simulink model "ac3_example_MMCT"  (R2023a)
settings: Solver=FixedStepDiscrete  StartTime=0.0  StopTime=3  FixedStep=Ts  RelTol=1e-3  EnableMultiTasking=on
PreLoadFcn:
  | Ts = 2e-6;
undefined symbols (not defined in the file): DiscIntNeverNeededParam
libraries: simulink_extras x7, spsCurrentMeasurementLib x3, spsVoltageMeasurementLib x3, spsDrivesPrivateModels x2, spsStairGeneratorLib x2, spsThreePhaseSourceLib x1, spsDrivesDcBusModel x1, spsSpaceVectorModulatorLib x1, eeAdaptiveController x1, slctrlblks x1, simulink x1, slpidlib x1
(part 2 of 3)

== system ac3_example_MMCT/Field-Oriented Control Induction Motor Drive/F.O.C./Average/Teta Calculation ==
  note: wm= Rotor mechanical speed (rad/s)
  note: wr = Rotor frequency (rad/s) = Lm *Iq / ( Tr * Phir)
  note: Teta= Electrical angle= integ ( wr + wm)
  Iq : Inport
  Phir : Inport  Port=2
  wm : Inport  Port=3
  Discrete-Time Integrator : DiscreteIntegrator  IntegratorMethod=Integration: Trapezoidal  SampleTime=Tvect  ICPrevOutput=DiscIntNeverNeededParam  ICPrevScaledInput=DiscIntNeverNeededParam
  Fcn : Fcn  Expr=Lm*u[1]/(u[2]*(Lr/Rr))
  Gain2 : Gain  SaturateOnIntegerOverflow=on  OutDataTypeStr=Inherit: Same as input  ParamDataTypeStr=Inherit: Same as input
  Gain3 : Gain  Gain=p  SaturateOnIntegerOverflow=on  OutDataTypeStr=Inherit: Same as input  ParamDataTypeStr=Inherit: Same as input
  Mux : Mux  Inputs=2
  Saturation : Saturate  UpperLimit=inf  LowerLimit=1e-3
  Sum : Sum  InputSameDT=on  SaturateOnIntegerOverflow=on  OutDataTypeStr=Inherit: Same as first input
  Unit Delay5 : UnitDelay  SampleTime=Tvect  HasFrameUpgradeWarning=on
  Thetae : Outport  InitialOutput=0  VectorParamsAs1DForOutWhenUnconnected=off
  we : Outport  Port=2  InitialOutput=0  VectorParamsAs1DForOutWhenUnconnected=off
  wires:
  Fcn/1 -> Gain2/1
  wm/1 -> Gain3/1
  Gain2/1 -> Sum/1
  Gain3/1 -> Sum/2
  Sum/1 -> we/1, Discrete-Time Integrator/1
  Discrete-Time Integrator/1 -> Thetae/1
  Unit Delay5/1 -> Mux/1
  Saturation/1 -> Mux/2
  Mux/1 -> Fcn/1
  Iq/1 -> Unit Delay5/1
  Phir/1 -> Saturation/1

== system ac3_example_MMCT/Field-Oriented Control Induction Motor Drive/F.O.C./Average/id* Calculation ==
  note: Lm= 34.7 mH
  note: Id* = Phir*/ Lm
  Phir* : Inport
  KF : Gain  Gain=1/Lm  SaturateOnIntegerOverflow=on  OutDataTypeStr=Inherit: Same as input  ParamDataTypeStr=Inherit: Same as input
  Id* : Outport  VectorParamsAs1DForOutWhenUnconnected=off
  wires:
  Phir*/1 -> KF/1
  KF/1 -> Id*/1

== system ac3_example_MMCT/Field-Oriented Control Induction Motor Drive/F.O.C./Average/iqs* Calculation ==
  Te* : Inport
  Phir : Inport  Port=2
  Fcn : Fcn  Expr=(2/3)*(1/p)*(Lr/Lm)*u[1]/(u[2]+1e-3*0)
  Mux1 : Mux  Inputs=2
  Saturation : Saturate  UpperLimit=inf  LowerLimit=1e-3
  Iq* : Outport  InitialOutput=0  VectorParamsAs1DForOutWhenUnconnected=off
  wires:
  Saturation/1 -> Mux1/2
  Mux1/1 -> Fcn/1
  Te*/1 -> Mux1/1
  Fcn/1 -> Iq*/1
  Phir/1 -> Saturation/1

== system ac3_example_MMCT/Field-Oriented Control Induction Motor Drive/F.O.C./Detailed/ABC-DQ ==
  Teta : Inport
  Iabc : Inport  Port=2
  Fcn : Fcn  Expr=sin(u)
  Fcn1 : Fcn  Expr=cos(u)
  Gain : Gain  Gain=2/3  SaturateOnIntegerOverflow=on  OutDataTypeStr=Inherit: Same as input  ParamDataTypeStr=Inherit: Same as input
  Gain1 : Gain  Gain=2/3  SaturateOnIntegerOverflow=on  OutDataTypeStr=Inherit: Same as input  ParamDataTypeStr=Inherit: Same as input
  Mux : Mux  Inputs=[1 1 3]
  id : Fcn  Expr=u[1]*u[3]+(1.7320508*u[2]-u[1])*u[4]*0.5+(-u[1]-1.7320508*u[2])*u[5]*0.5
  iq : Fcn  Expr=-u[2]*u[3]+(u[2]+1.7320508*u[1])*u[4]*0.5+(u[2]-1.7320508*u[1])*u[5]*0.5
  Id : Outport  InitialOutput=0  VectorParamsAs1DForOutWhenUnconnected=off
  Iq : Outport  Port=2  InitialOutput=0  VectorParamsAs1DForOutWhenUnconnected=off
  wires:
  Gain1/1 -> Iq/1
  Gain/1 -> Id/1
  id/1 -> Gain/1
  iq/1 -> Gain1/1
  Iabc/1 -> Mux/3
  Mux/1 -> id/1, iq/1
  Teta/1 -> Fcn/1, Fcn1/1
  Fcn1/1 -> Mux/1
  Fcn/1 -> Mux/2

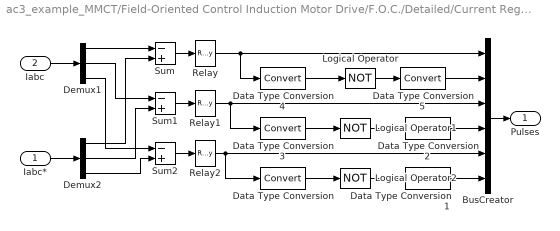
== system ac3_example_MMCT/Field-Oriented Control Induction Motor Drive/F.O.C./Detailed/Current Regulator ==
  Iabc* : Inport
  Iabc : Inport  Port=2
  BusCreator : BusCreator  Inputs=6
  Data Type Conversion{,1..5} (6 alike) : DataTypeConversion
  Demux1 : Demux  Outputs=3
      settings: DisplayOption=none
  Demux2 : Demux  Outputs=3
      settings: DisplayOption=none
  Logical Operator : Logic  Operator=NOT
  Logical Operator1 : Logic  Operator=NOT
  Logical Operator2 : Logic  Operator=NOT
  Relay : Relay  OnSwitchValue=h/2  OffSwitchValue=-h/2
  Relay1 : Relay  OnSwitchValue=h/2  OffSwitchValue=-h/2
  Relay2 : Relay  OnSwitchValue=h/2  OffSwitchValue=-h/2
  Sum : Sum  Inputs=-+  InputSameDT=on  SaturateOnIntegerOverflow=on  OutDataTypeStr=Inherit: Same as first input
  Sum1 : Sum  Inputs=-+  InputSameDT=on  SaturateOnIntegerOverflow=on  OutDataTypeStr=Inherit: Same as first input
  Sum2 : Sum  Inputs=-+  InputSameDT=on  SaturateOnIntegerOverflow=on  OutDataTypeStr=Inherit: Same as first input
  Pulses : Outport  InitialOutput=0  VectorParamsAs1DForOutWhenUnconnected=off
  wires:
  Logical Operator2/1 -> Data Type Conversion1/1
  Logical Operator1/1 -> Data Type Conversion2/1
  Logical Operator/1 -> Data Type Conversion5/1
  Relay2/1 -> BusCreator/5, Data Type Conversion/1
  Relay1/1 -> BusCreator/3, Data Type Conversion3/1
  Relay/1 -> BusCreator/1, Data Type Conversion4/1
  Iabc*/1 -> Demux2/1
  Demux2/1 -> Sum/2
  Demux2/2 -> Sum1/2
  Demux2/3 -> Sum2/2
  Demux1/3 -> Sum2/1
  Sum2/1 -> Relay2/1
  Iabc/1 -> Demux1/1
  BusCreator/1 -> Pulses/1
  Demux1/2 -> Sum1/1
  Demux1/1 -> Sum/1
  Sum1/1 -> Relay1/1
  Sum/1 -> Relay/1
  Data Type Conversion/1 -> Logical Operator2/1
  Data Type Conversion1/1 -> BusCreator/6
  Data Type Conversion2/1 -> BusCreator/4
  Data Type Conversion3/1 -> Logical Operator1/1
  Data Type Conversion4/1 -> Logical Operator/1
  Data Type Conversion5/1 -> BusCreator/2

== system ac3_example_MMCT/Field-Oriented Control Induction Motor Drive/F.O.C./Detailed/DQ-ABC ==
  Id* : Inport
  Iq* : Inport  Port=2
  Teta : Inport  Port=3
  Fcn : Fcn  Expr=sin(u)
  Fcn1 : Fcn  Expr=cos(u)
  Gain2 : Gain  SaturateOnIntegerOverflow=on  OutDataTypeStr=Inherit: Same as input  ParamDataTypeStr=Inherit: Same as input
  Gain3 : Gain  SaturateOnIntegerOverflow=on  OutDataTypeStr=Inherit: Same as input  ParamDataTypeStr=Inherit: Same as input
  Gain4 : Gain  SaturateOnIntegerOverflow=on  OutDataTypeStr=Inherit: Same as input  ParamDataTypeStr=Inherit: Same as input
  Mux : Mux
  Mux2 : Mux  Inputs=3
  ia : Fcn  Expr=-u[3]*u[2] + u[4]*u[1]
  ib : Fcn  Expr=(-u[1]+1.7320508*u[2])*u[4]*0.5+(u[2]+1.7320508*u[1])*u[3]*0.5
  ic : Sum  Inputs=--  InputSameDT=on  SaturateOnIntegerOverflow=on  OutDataTypeStr=Inherit: Same as first input
  Iabc* : Outport  InitialOutput=0  VectorParamsAs1DForOutWhenUnconnected=off
  wires:
  ib/1 -> ic/1, Gain3/1
  ia/1 -> ic/2, Gain2/1
  Gain2/1 -> Mux2/1
  Gain4/1 -> Mux2/3
  ic/1 -> Gain4/1
  Gain3/1 -> Mux2/2
  Id*/1 -> Mux/4
  Iq*/1 -> Mux/3
  Teta/1 -> Fcn/1, Fcn1/1
  Mux/1 -> ia/1, ib/1
  Mux2/1 -> Iabc*/1
  Fcn1/1 -> Mux/1
  Fcn/1 -> Mux/2

== system ac3_example_MMCT/Field-Oriented Control Induction Motor Drive/F.O.C./Detailed/Flux Calculation ==
  note: Phir = Lm *Id / (1 +Tr .s)
  Id : Inport
  Discrete Transfer Fcn1 : DiscreteTransferFcn  Numerator=[1-exp(-(Rr/(Lr))*Tvect)]  Denominator=[1 -exp(-(Rr/(Lr))*Tvect)]  SampleTime=Tvect
  Lm : Gain  Gain=Lm  SaturateOnIntegerOverflow=on  OutDataTypeStr=Inherit: Same as input  ParamDataTypeStr=Inherit: Same as input
  Phir : Outport  VectorParamsAs1DForOutWhenUnconnected=off
  wires:
  Lm/1 -> Discrete Transfer Fcn1/1
  Id/1 -> Lm/1
  Discrete Transfer Fcn1/1 -> Phir/1

== system ac3_example_MMCT/Field-Oriented Control Induction Motor Drive/F.O.C./Detailed/Flux_PI ==
  m_Flux : Inport
  Flux* : Inport  Port=2
  Discrete Transfer Fcn1 : DiscreteTransferFcn  Numerator=[1-exp(-(2*pi*fc)*Tvect)]  Denominator=[1 -exp(-(2*pi*fc)*Tvect)]  SampleTime=Tvect
  Discrete-Time Integrator : DiscreteIntegrator  IntegratorMethod=Integration: Trapezoidal  SampleTime=Tvect  LimitOutput=on  UpperSaturationLimit=csat(2)  LowerSaturationLimit=csat(1)  ICPrevOutput=DiscIntNeverNeededParam  ICPrevScaledInput=DiscIntNeverNeededParam
  Ki1 : Gain  Gain=ki  SaturateOnIntegerOverflow=on  OutDataTypeStr=Inherit: Same as input  ParamDataTypeStr=Inherit: Same as input
  Kp : Gain  Gain=kp  SaturateOnIntegerOverflow=on  OutDataTypeStr=Inherit: Same as input  ParamDataTypeStr=Inherit: Same as input
  Saturation : Saturate  UpperLimit=csat(2)  LowerLimit=csat(1)
  Sum : Sum  Inputs=|+-  SaturateOnIntegerOverflow=on
  Sum1 : Sum  Inputs=|++  SaturateOnIntegerOverflow=on
  Phir* : Outport  VectorParamsAs1DForOutWhenUnconnected=off
  wires:
  Ki1/1 -> Discrete-Time Integrator/1
  m_Flux/1 -> Discrete Transfer Fcn1/1
  Saturation/1 -> Phir*/1
  Flux*/1 -> Sum/1
  Discrete Transfer Fcn1/1 -> Sum/2
  Sum1/1 -> Saturation/1
  Kp/1 -> Sum1/2
  Discrete-Time Integrator/1 -> Sum1/1
  Sum/1 -> Ki1/1, Kp/1

== system ac3_example_MMCT/Field-Oriented Control Induction Motor Drive/F.O.C./Detailed/M_vector ==
  Constant1 : Constant  Value=[1 0 1 0 1 0]
  Constant3 : Constant  Value=[1 0 0 1 1 0]
  Pulse Generator1 : DiscretePulseGenerator  Period=8  PulseWidth=2  SampleTime=Tvect
  Switch1 : Switch  Threshold=0.5  InputSameDT=off
  Zero-Order Hold8 : ZeroOrderHold  SampleTime=Tvect
  vector : Outport  VectorParamsAs1DForOutWhenUnconnected=off
  wires:
  Switch1/1 -> vector/1
  Zero-Order Hold8/1 -> Switch1/2
  Pulse Generator1/1 -> Zero-Order Hold8/1
  Constant1/1 -> Switch1/3
  Constant3/1 -> Switch1/1

== system ac3_example_MMCT/Field-Oriented Control Induction Motor Drive/F.O.C./Detailed/Magnetisation ==
  Est_Flux : Inport
  Constant : Constant  Value=in_flux
  Constant1 : Constant  Value=0
  Data Type Conversion5 : DataTypeConversion
  Relational Operator : RelationalOperator  InputSameDT=off
  S-R Flip-Flop : simulink_extras/Flip Flops/S-R Flip-Flop  initial_condition=0
  Terminator : Terminator
  Zero-Order Hold5 : ZeroOrderHold  SampleTime=Tvect
  Start : Outport  VectorParamsAs1DForOutWhenUnconnected=off
  wires:
  Zero-Order Hold5/1 -> Relational Operator/2
  S-R Flip-Flop/2 -> Terminator/1
  S-R Flip-Flop/1 -> Start/1
  Constant1/1 -> Data Type Conversion5/1
  Constant/1 -> Zero-Order Hold5/1
  Relational Operator/1 -> S-R Flip-Flop/1
  Est_Flux/1 -> Relational Operator/1
  Data Type Conversion5/1 -> S-R Flip-Flop/2

== system ac3_example_MMCT/Field-Oriented Control Induction Motor Drive/F.O.C./Detailed/Switching control ==
  Pulses : Inport
  Control 1-2 : Subsystem
  Control 3-4 : Subsystem
  Control 5-6 : Subsystem
  Demux : Demux  Outputs=6
      settings: DisplayOption=none
  Mux : Mux  Inputs=6
  RF Pulses : Outport  VectorParamsAs1DForOutWhenUnconnected=off
  wires:
  Pulses/1 -> Demux/1
  Mux/1 -> RF Pulses/1
  Demux/1 -> Control 1-2/1(S)
  Demux/2 -> Control 1-2/2(!S)
  Demux/3 -> Control 3-4/1(S)
  Demux/4 -> Control 3-4/2(!S)
  Demux/5 -> Control 5-6/1(S)
  Demux/6 -> Control 5-6/2(!S)
  Control 1-2/1(S_Limited) -> Mux/1
  Control 1-2/2(!S_Limited) -> Mux/2
  Control 3-4/1(S_Limited) -> Mux/3
  Control 3-4/2(!S_Limited) -> Mux/4
  Control 5-6/1(S_Limited) -> Mux/5
  Control 5-6/2(!S_Limited) -> Mux/6

== system ac3_example_MMCT/Field-Oriented Control Induction Motor Drive/F.O.C./Detailed/Teta Calculation ==
  note: wm= Rotor mechanical speed (rad/s)
  note: wr = Rotor frequency (rad/s) = Lm *Iq / ( Tr * Phir)
  note: Teta= Electrical angle= integ ( wr + wm)
  Iq : Inport
  Phir : Inport  Port=2
  wm : Inport  Port=3
  Discrete-Time Integrator : DiscreteIntegrator  IntegratorMethod=Integration: Trapezoidal  SampleTime=Tvect  ICPrevOutput=DiscIntNeverNeededParam  ICPrevScaledInput=DiscIntNeverNeededParam
  Fcn : Fcn  Expr=Lm*u[1]/(u[2]*(Lr/Rr)+1e-3*0)
  Gain2 : Gain  SaturateOnIntegerOverflow=on  OutDataTypeStr=Inherit: Same as input  ParamDataTypeStr=Inherit: Same as input
  Gain3 : Gain  Gain=p  SaturateOnIntegerOverflow=on  OutDataTypeStr=Inherit: Same as input  ParamDataTypeStr=Inherit: Same as input
  Mux : Mux  Inputs=2
  Saturation : Saturate  UpperLimit=inf  LowerLimit=1e-3
  Sum : Sum  InputSameDT=on  SaturateOnIntegerOverflow=on  OutDataTypeStr=Inherit: Same as first input
  Unit Delay5 : UnitDelay  SampleTime=Tvect  HasFrameUpgradeWarning=on
  Teta : Outport  InitialOutput=0  VectorParamsAs1DForOutWhenUnconnected=off
  wires:
  Unit Delay5/1 -> Mux/1
  Saturation/1 -> Mux/2
  Mux/1 -> Fcn/1
  Iq/1 -> Unit Delay5/1
  Phir/1 -> Saturation/1
  Fcn/1 -> Gain2/1
  wm/1 -> Gain3/1
  Gain2/1 -> Sum/1
  Gain3/1 -> Sum/2
  Sum/1 -> Discrete-Time Integrator/1
  Discrete-Time Integrator/1 -> Teta/1

== system ac3_example_MMCT/Field-Oriented Control Induction Motor Drive/F.O.C./Detailed/id* Calculation ==
  note: Lm= 34.7 mH
  note: Id* = Phir*/ Lm
  Phir* : Inport
  KF : Gain  Gain=1/Lm  SaturateOnIntegerOverflow=on  OutDataTypeStr=Inherit: Same as input  ParamDataTypeStr=Inherit: Same as input
  Id* : Outport  VectorParamsAs1DForOutWhenUnconnected=off
  wires:
  Phir*/1 -> KF/1
  KF/1 -> Id*/1

== system ac3_example_MMCT/Field-Oriented Control Induction Motor Drive/F.O.C./Detailed/iqs* Calculation ==
  Te* : Inport
  Phir : Inport  Port=2
  Fcn : Fcn  Expr=(2/3)*(1/p)*(Lr/Lm)*u[1]/(u[2]+1e-3*0)
  Mux1 : Mux  Inputs=2
  Saturation : Saturate  UpperLimit=inf  LowerLimit=1e-3
  Iq* : Outport  InitialOutput=0  VectorParamsAs1DForOutWhenUnconnected=off
  wires:
  Saturation/1 -> Mux1/2
  Mux1/1 -> Fcn/1
  Te*/1 -> Mux1/1
  Fcn/1 -> Iq*/1
  Phir/1 -> Saturation/1

== system ac3_example_MMCT/Field-Oriented Control Induction Motor Drive/F.O.C./Detailed SVM/ABC-DQ1 ==
  Theta : Inport
  Iabc : Inport  Port=2
  Fcn : Fcn  Expr=sin(u)
  Fcn1 : Fcn  Expr=cos(u)
  Gain : Gain  Gain=2/3  SaturateOnIntegerOverflow=on  OutDataTypeStr=Inherit: Same as input  ParamDataTypeStr=Inherit: Same as input
  Gain1 : Gain  Gain=2/3  SaturateOnIntegerOverflow=on  OutDataTypeStr=Inherit: Same as input  ParamDataTypeStr=Inherit: Same as input
  Mux : Mux  Inputs=[1 1 3]
  id : Fcn  Expr=u[2]*u[3]+(-u[2]-1.7320508*u[1])*u[4]*0.5+(-u[2]+1.7320508*u[1])*u[5]*0.5
  iq : Fcn  Expr=u[1]*u[3]+(1.7320508*u[2]-u[1]) *u[4]*0.5+(-u[1]-1.7320508*u[2])*u[5]*0.5
  Id : Outport  InitialOutput=0  VectorParamsAs1DForOutWhenUnconnected=off
  Iq : Outport  Port=2  InitialOutput=0  VectorParamsAs1DForOutWhenUnconnected=off
  wires:
  Fcn/1 -> Mux/2
  Fcn1/1 -> Mux/1
  Theta/1 -> Fcn1/1, Fcn/1
  Mux/1 -> iq/1, id/1
  Iabc/1 -> Mux/3
  iq/1 -> Gain1/1
  id/1 -> Gain/1
  Gain/1 -> Id/1
  Gain1/1 -> Iq/1

== system ac3_example_MMCT/Field-Oriented Control Induction Motor Drive/F.O.C./Detailed SVM/Flux Calculation ==
  note: 公式不懂
  note: Phir = Lm *Id / (1 +Tr .s)
  Id : Inport
  Discrete Transfer Fcn1 : DiscreteTransferFcn  Numerator=[1-exp(-(Rr/(Lr))*Tvect)]  Denominator=[1 -exp(-(Rr/(Lr))*Tvect)]  SampleTime=Tvect
  Lm : Gain  Gain=Lm  SaturateOnIntegerOverflow=on  OutDataTypeStr=Inherit: Same as input  ParamDataTypeStr=Inherit: Same as input
  Scope : Scope
  Phir : Outport  VectorParamsAs1DForOutWhenUnconnected=off
  wires:
  Lm/1 -> Discrete Transfer Fcn1/1
  Id/1 -> Lm/1
  Discrete Transfer Fcn1/1 -> Phir/1, Scope/1

== system ac3_example_MMCT/Field-Oriented Control Induction Motor Drive/F.O.C./Detailed SVM/Flux_PI ==
  m_Flux : Inport
  Flux* : Inport  Port=2
  Discrete Transfer Fcn1 : DiscreteTransferFcn  Numerator=[1-exp(-(2*pi*fc)*Tvect)]  Denominator=[1 -exp(-(2*pi*fc)*Tvect)]  SampleTime=Tvect
  Discrete-Time Integrator : DiscreteIntegrator  IntegratorMethod=Integration: Trapezoidal  SampleTime=Tvect  LimitOutput=on  UpperSaturationLimit=csat(2)  LowerSaturationLimit=csat(1)  ICPrevOutput=DiscIntNeverNeededParam  ICPrevScaledInput=DiscIntNeverNeededParam
  Ki1 : Gain  Gain=ki  SaturateOnIntegerOverflow=on  OutDataTypeStr=Inherit: Same as input  ParamDataTypeStr=Inherit: Same as input
  Kp : Gain  Gain=kp  SaturateOnIntegerOverflow=on  OutDataTypeStr=Inherit: Same as input  ParamDataTypeStr=Inherit: Same as input
  Saturation : Saturate  UpperLimit=csat(2)  LowerLimit=csat(1)
  Sum : Sum  Inputs=|+-  SaturateOnIntegerOverflow=on
  Sum1 : Sum  Inputs=|++  SaturateOnIntegerOverflow=on
  Phir* : Outport  VectorParamsAs1DForOutWhenUnconnected=off
  wires:
  Ki1/1 -> Discrete-Time Integrator/1
  m_Flux/1 -> Discrete Transfer Fcn1/1
  Saturation/1 -> Phir*/1
  Flux*/1 -> Sum/1
  Discrete Transfer Fcn1/1 -> Sum/2
  Sum1/1 -> Saturation/1
  Kp/1 -> Sum1/2
  Discrete-Time Integrator/1 -> Sum1/1
  Sum/1 -> Ki1/1, Kp/1

== system ac3_example_MMCT/Field-Oriented Control Induction Motor Drive/F.O.C./Detailed SVM/Id_PI regulator ==
  Id* : Inport
  Id : Inport  Port=2
  Discrete-Time Integrator : DiscreteIntegrator  IntegratorMethod=Integration: Trapezoidal  SampleTime=Tvect  LimitOutput=on  UpperSaturationLimit=1  LowerSaturationLimit=-1  ICPrevOutput=DiscIntNeverNeededParam  ICPrevScaledInput=DiscIntNeverNeededParam
  Ki : Gain  Gain=ki_Id  SaturateOnIntegerOverflow=on  OutDataTypeStr=Inherit: Same as input  ParamDataTypeStr=Inherit: Same as input
  Kp : Gain  Gain=kp_Id  SaturateOnIntegerOverflow=on  OutDataTypeStr=Inherit: Same as input  ParamDataTypeStr=Inherit: Same as input
  Saturation : Saturate  UpperLimit=inf  LowerLimit=-inf
  Sum : Sum  Inputs=|+-  SaturateOnIntegerOverflow=on
  Sum1 : Sum  Inputs=|++  SaturateOnIntegerOverflow=on
  Vds* : Outport  VectorParamsAs1DForOutWhenUnconnected=off
  wires:
  Sum/1 -> Kp/1, Discrete-Time Integrator/1
  Discrete-Time Integrator/1 -> Ki/1
  Ki/1 -> Sum1/1
  Kp/1 -> Sum1/2
  Sum1/1 -> Saturation/1
  Id*/1 -> Sum/1
  Saturation/1 -> Vds*/1
  Id/1 -> Sum/2

== system ac3_example_MMCT/Field-Oriented Control Induction Motor Drive/F.O.C./Detailed SVM/Iq-PI regulator ==
  Iq* : Inport
  Iq : Inport  Port=2
  Discrete-Time Integrator : DiscreteIntegrator  IntegratorMethod=Integration: Trapezoidal  SampleTime=Tvect  LimitOutput=on  UpperSaturationLimit=1  LowerSaturationLimit=-1  ICPrevOutput=DiscIntNeverNeededParam  ICPrevScaledInput=DiscIntNeverNeededParam
  Ki : Gain  Gain=ki_Iq  SaturateOnIntegerOverflow=on  OutDataTypeStr=Inherit: Same as input  ParamDataTypeStr=Inherit: Same as input
  Kp : Gain  Gain=kp_Iq  SaturateOnIntegerOverflow=on  OutDataTypeStr=Inherit: Same as input  ParamDataTypeStr=Inherit: Same as input
  Saturation : Saturate  UpperLimit=inf  LowerLimit=-inf
  Sum : Sum  Inputs=|+-  SaturateOnIntegerOverflow=on
  Sum1 : Sum  Inputs=|++  SaturateOnIntegerOverflow=on
  Vqs* : Outport  VectorParamsAs1DForOutWhenUnconnected=off
  wires:
  Iq/1 -> Sum/2
  Saturation/1 -> Vqs*/1
  Iq*/1 -> Sum/1
  Sum1/1 -> Saturation/1
  Kp/1 -> Sum1/2
  Ki/1 -> Sum1/1
  Discrete-Time Integrator/1 -> Ki/1
  Sum/1 -> Kp/1, Discrete-Time Integrator/1

== system ac3_example_MMCT/Field-Oriented Control Induction Motor Drive/F.O.C./Detailed SVM/M_vector ==
  Constant1 : Constant  Value=[1 0 1 0 1 0]
  Constant3 : Constant  Value=[1 0 0 1 1 0]
  Pulse Generator1 : DiscretePulseGenerator  Period=8  PulseWidth=2  SampleTime=Tvect
  Rate Transition3 : RateTransition
  Switch1 : Switch  Threshold=0.5  InputSameDT=off
  Zero-Order Hold8 : ZeroOrderHold  SampleTime=Tvect
  vector : Outport  VectorParamsAs1DForOutWhenUnconnected=off
  wires:
  Switch1/1 -> vector/1
  Pulse Generator1/1 -> Zero-Order Hold8/1
  Constant1/1 -> Switch1/3
  Constant3/1 -> Switch1/1
  Zero-Order Hold8/1 -> Rate Transition3/1
  Rate Transition3/1 -> Switch1/2

== system ac3_example_MMCT/Field-Oriented Control Induction Motor Drive/F.O.C./Detailed SVM/Magnetisation ==
  Est_Flux : Inport
  Constant : Constant  Value=in_flux
  Constant1 : Constant  Value=0
  Data Type Conversion5 : DataTypeConversion
  Relational Operator : RelationalOperator  InputSameDT=off
  S-R Flip-Flop : simulink_extras/Flip Flops/S-R Flip-Flop  initial_condition=0
  Terminator : Terminator
  Zero-Order Hold5 : ZeroOrderHold  SampleTime=Tvect
  Start : Outport  VectorParamsAs1DForOutWhenUnconnected=off
  wires:
  Zero-Order Hold5/1 -> Relational Operator/2
  S-R Flip-Flop/2 -> Terminator/1
  S-R Flip-Flop/1 -> Start/1
  Constant1/1 -> Data Type Conversion5/1
  Constant/1 -> Zero-Order Hold5/1
  Relational Operator/1 -> S-R Flip-Flop/1
  Est_Flux/1 -> Relational Operator/1
  Data Type Conversion5/1 -> S-R Flip-Flop/2

== system ac3_example_MMCT/Field-Oriented Control Induction Motor Drive/F.O.C./Detailed SVM/Subsystem1 ==
  note: 确定电压象限后计算相邻电压矢量的作用时间
  note: 确定矢量的象限
  Angle : Inport
  ab : Inport  Port=2
  Vdc_bus : Inport  Port=3
  Mux : Mux  Inputs=2
  Rate Transition : RateTransition
  Rate Transition4 : RateTransition
  Scope : Scope
  Zero-Order Hold6 : ZeroOrderHold  SampleTime=Ts
  Zero-Order Hold7 : ZeroOrderHold  SampleTime=Ts
  ab vector sector : Subsystem
  gates logic1 : Subsystem
  ramp generator : spsSpaceVectorModulatorLib/Space Vector Modulator/Detailed/ramp generator  SystemSampleTime=-1  VariantActivationTime=update diagram  Latency=0  AutoFrameSizeCalculation=off
  switching time calculator : Subsystem
  gate_signals : Outport  VectorParamsAs1DForOutWhenUnconnected=off
  wires:
  ramp generator/1 -> gates logic1/1(ramp)
  ramp generator/2 -> switching time calculator/1(Trig)
  switching time calculator/1(Gate timing) -> gates logic1/2(gate_timing)
  gates logic1/1(gates_signals) -> gate_signals/1
  Angle/1 -> ab vector sector/1(Angle)
  ab vector sector/1(Sector) -> Rate Transition/1
  Rate Transition4/1 -> Zero-Order Hold7/1
  Rate Transition/1 -> Zero-Order Hold6/1
  Zero-Order Hold7/1 -> switching time calculator/3(a_b_vbus)
  Zero-Order Hold6/1 -> switching time calculator/2(Sector)
  ab/1 -> Mux/1
  Vdc_bus/1 -> Mux/2
  Mux/1 -> Scope/1, Rate Transition4/1

== system ac3_example_MMCT/Field-Oriented Control Induction Motor Drive/F.O.C./Detailed SVM/Subsystem2 ==
  Usa : Inport
  Usb : Inport  Port=2
  Isa : Inport  Port=3
  Isb : Inport  Port=4
  Wr : Inport  Port=5
  Demux : Demux
  Model Reference Adaptive Controller : eeAdaptiveController/Model Reference Adaptive Controller  Kp=1  Ki=1  Kd=0  Kaw=1  UseFilter=off  N=100  up=5  lo=-5  Ts=-1  TfType=Discrete-time  numd=[0.01 -0.0099]  dend=[1 -1.9801 0.9802]  numc=[1 1]  denc=[1 2 1]  Tsd=0.01  gamma=0.5
      settings: LibrarySourceBlock=|
      | ee_sl_lib/General Control/Model Reference
      | Adaptive Controller
  Model Reference Adaptive Control : slctrlblks/Model Reference Adaptive Control  selectType=Direct  A=0  B=1  Ahat=0  ALrEnable=on  gamma_a=1  ALrEnableMod=on  Bhat=1  BLrEnable=on  gamma_b=1  BLrEnableMod=on  externalKtauEnable=off  k_tau=-1  estParamOutput=off  Am=-1  Bm=1  kx=0  FBLrEnable=on  gamma_kx=1  FBLrEnableMod=on  kr=0  FFLrEnable=on  gamma_kr=1  FFLrEnableMod=on  AdaptEnable=on  gamma=1  WLrEnableMod=on  Q=1  FeatureTypeOptions=State  shlHiddenLayerSize=10  gamma_V=0.1  nCen=20  cSpanMin=-1  cSpanMax=1  cSig=5  adaptiveCntrlOutport=off  modChoice=None  sigma_val=0.1
      settings: LibrarySourceBlock=slctrlblks/SHL Model Reference Adaptive Control
  Mux : Mux  Inputs=6
  S-Function : S-Function  FunctionName=MRAS  Parameters=Lm,Lr,Ls,Sigma,tao  SFunctionDeploymentMode=off  EnableBusSupport=off
  S-Function Examples : simulink/User-Defined Functions/S-Function Examples
  Subsystem : Subsystem
  Pra1 : Outport
  Prb1 : Outport  Port=2
  wires:
  Subsystem/1(Tr) -> Mux/6
  S-Function/1 -> Demux/1
  Usa/1 -> Mux/1
  Wr/1 -> Mux/5
  Demux/3 -> Subsystem/2(Q1)
  Mux/1 -> S-Function/1
  Demux/4 -> Subsystem/1(Q)
  Demux/2 -> Prb1/1  "Prb1"
  Isa/1 -> Mux/3
  Usb/1 -> Mux/2
  Isb/1 -> Mux/4
  Demux/1 -> Pra1/1  "Pra1"

== system ac3_example_MMCT/Field-Oriented Control Induction Motor Drive/F.O.C./Detailed SVM/Theta Calculation ==
  note: 这个公式不懂
  note: 这三个式子说明是转子磁场定向控制
  note: wm= Rotor mechanical speed (rad/s)
  note: wr = Rotor frequency (rad/s) = Lm *Iq / ( Tr * Phir)
  note: Teta= Electrical angle= integ ( wr + wm)
  Iq : Inport
  Phir : Inport  Port=2
  wm : Inport  Port=3
  Discrete-Time Integrator : DiscreteIntegrator  IntegratorMethod=Integration: Trapezoidal  SampleTime=Tvect  ICPrevOutput=DiscIntNeverNeededParam  ICPrevScaledInput=DiscIntNeverNeededParam
  Fcn : Fcn  Expr=Lm*u[1]/(u[2]*(Lr/Rr)+1e-3*0)
  Gain2 : Gain  SaturateOnIntegerOverflow=on  OutDataTypeStr=Inherit: Same as input  ParamDataTypeStr=Inherit: Same as input
  Gain3 : Gain  Gain=p  SaturateOnIntegerOverflow=on  OutDataTypeStr=Inherit: Same as input  ParamDataTypeStr=Inherit: Same as input
  Mux : Mux  Inputs=2
  Saturation : Saturate  UpperLimit=inf  LowerLimit=1e-3
  Scope : Scope
  Sum : Sum  InputSameDT=on  SaturateOnIntegerOverflow=on  OutDataTypeStr=Inherit: Same as first input
  Unit Delay5 : UnitDelay  SampleTime=Tvect  HasFrameUpgradeWarning=on
  Theta : Outport  InitialOutput=0  VectorParamsAs1DForOutWhenUnconnected=off
  wires:
  Unit Delay5/1 -> Mux/1
  Saturation/1 -> Mux/2
  Mux/1 -> Fcn/1
  Iq/1 -> Unit Delay5/1
  Phir/1 -> Saturation/1
  Fcn/1 -> Gain2/1
  wm/1 -> Gain3/1
  Gain2/1 -> Sum/1
  Gain3/1 -> Sum/2
  Sum/1 -> Discrete-Time Integrator/1
  Discrete-Time Integrator/1 -> Scope/1, Theta/1

== system ac3_example_MMCT/Field-Oriented Control Induction Motor Drive/F.O.C./Detailed SVM/dq//ab1 ==
  note: 静止三相坐标系到静止两相坐标系的转换
  Vqs* : Inport
  Vds* : Inport  Port=2
  Theta : Inport  Port=3
  DQ-ABC : Subsystem
      mask Display:
      | port_label('input',1,'Vqs*')
      | port_label('input',2,'Vds*')
      | port_label('input',3,'{\theta}','texmode','on')
      | port_label('output',1,'Vabc*')
  ab transform : Subsystem
  Angle : Outport  VectorParamsAs1DForOutWhenUnconnected=off
  ab : Outport  Port=2  VectorParamsAs1DForOutWhenUnconnected=off
  wires:
  ab transform/2(ab) -> ab/1
  DQ-ABC/1(Vabc*) -> ab transform/1(Vabc)
  Vqs*/1 -> DQ-ABC/1(Vq*)
  ab transform/1(Angle) -> Angle/1
  Theta/1 -> DQ-ABC/3(Teta)
  Vds*/1 -> DQ-ABC/2(Vd*)

== system ac3_example_MMCT/Field-Oriented Control Induction Motor Drive/F.O.C./Detailed SVM/id* Calculation ==
  note: Lm= 34.7 mH
  note: Id* = Phir*/ Lm
  Phir* : Inport
  KF : Gain  Gain=1/Lm  SaturateOnIntegerOverflow=on  OutDataTypeStr=Inherit: Same as input  ParamDataTypeStr=Inherit: Same as input
  Id* : Outport  VectorParamsAs1DForOutWhenUnconnected=off
  wires:
  Phir*/1 -> KF/1
  KF/1 -> Id*/1

== system ac3_example_MMCT/Field-Oriented Control Induction Motor Drive/F.O.C./Detailed SVM/iqs* Calculation ==
  Te* : Inport
  Phir : Inport  Port=2
  Fcn : Fcn  Expr=(2/3)*(1/p)*(Lr/Lm)*u[1]/(u[2]+1e-3*0)
  Mux1 : Mux  Inputs=2
  Saturation : Saturate  UpperLimit=inf  LowerLimit=1e-3
  Iq* : Outport  InitialOutput=0  VectorParamsAs1DForOutWhenUnconnected=off
  wires:
  Saturation/1 -> Mux1/2
  Mux1/1 -> Fcn/1
  Te*/1 -> Mux1/1
  Fcn/1 -> Iq*/1
  Phir/1 -> Saturation/1

== system ac3_example_MMCT/Field-Oriented Control Induction Motor Drive/F.O.C./Detailed SVM/low pass bus filter ==
  Vbus : Inport
  Discrete Transfer Fcn1 : DiscreteTransferFcn  Numerator=[1-exp(-2*pi*fc_bus*Tvect)]  Denominator=[1 -exp(-2*pi*fc_bus*Tvect)]  SampleTime=Tvect
  Saturation : Saturate  UpperLimit=inf  LowerLimit=1
  FVbus : Outport  VectorParamsAs1DForOutWhenUnconnected=off
  wires:
  Saturation/1 -> FVbus/1
  Vbus/1 -> Discrete Transfer Fcn1/1
  Discrete Transfer Fcn1/1 -> Saturation/1

== system ac3_example_MMCT/Field-Oriented Control Induction Motor Drive/Speed Controller/Speed Controller (AC)/AC345 ==
  note: 根据给定转速来计算转矩磁通的标准值
  N : Inport
  N* : Inport  Port=2
  MagC : Inport  Port=3
  Abs : Abs
  Bus Creator3 : BusCreator  Inputs=4
  Flux table : DriveInternalModels/AC drives/Speed Controller AC345/Speed Controller/Flux table  SystemSampleTime=-1  VariantActivationTime=update diagram  Latency=0  AutoFrameSizeCalculation=off
  Product : Product  SaturateOnIntegerOverflow=on  OutDataTypeStr=Inherit: Same as first input
  Rate Transition1 : RateTransition
  Speed controller (generic AC) : Subsystem  AncestorBlock=spsDrivesSpeedControllerModel/Speed controller (generic AC)
      settings: LibrarySourceBlock=spsDrivesSpeedControllerModel/Speed controller (generic AC)
  Flux* : Outport  VectorParamsAs1DForOutWhenUnconnected=off
  Torque* : Outport  Port=2  VectorParamsAs1DForOutWhenUnconnected=off
  Ctrl : Outport  Port=3  VectorParamsAs1DForOutWhenUnconnected=off
  wires:
  Bus Creator3/1 -> Ctrl/1  "Ctrl"
  Speed controller (generic AC)/5(Ref) -> Bus Creator3/4
  Speed controller (generic AC)/4(error) -> Bus Creator3/3
  Speed controller (generic AC)/3(torque_ref) -> Bus Creator3/1
  Rate Transition1/1 -> Flux*/1  "Flux*"
  Product/1 -> Speed controller (generic AC)/1(Ref_in)
  Speed controller (generic AC)/2(Ref_out) -> Abs/1
  N/1 -> Speed controller (generic AC)/2(Meas)
  Speed controller (generic AC)/1(Torque*) -> Torque*/1
  N*/1 -> Product/1
  MagC/1 -> Product/2
  Abs/1 -> Flux table/1
  Flux table/1 -> Rate Transition1/1, Bus Creator3/2  "Flux reference (Wb)"

== system ac3_example_MMCT/Field-Oriented Control Induction Motor Drive/Speed Controller/Speed Controller (AC)/AC678 ==
  N : Inport
  N* : Inport  Port=2
  MagC : Inport  Port=3
  AC678 : Subsystem
  gnd1 : Ground
  term3 : Terminator
  Flux* : Outport  VectorParamsAs1DForOutWhenUnconnected=off
  Torque* : Outport  Port=2  VectorParamsAs1DForOutWhenUnconnected=off
  Ctrl : Outport  Port=3  VectorParamsAs1DForOutWhenUnconnected=off
  wires:
  gnd1/1 -> Flux*/1
  MagC/1 -> term3/1
  AC678/2(Ctrl) -> Ctrl/1
  AC678/1(Torque*) -> Torque*/1
  N/1 -> AC678/1(N)
  N*/1 -> AC678/2(N*)

== system ac3_example_MMCT/Field-Oriented Control Induction Motor Drive/F.O.C./Detailed/Switching control/Control 1-2 ==
  S : Inport
  !S : Inport  Port=2
  Data Type Conversion2 : DataTypeConversion  OutDataTypeStr=boolean  SaturateOnIntegerOverflow=off  RndMeth=Floor
  Data Type Conversion8 : DataTypeConversion  OutDataTypeStr=boolean  SaturateOnIntegerOverflow=off  RndMeth=Floor
  Product2 : Product  RndMeth=Zero
  Product3 : Product  RndMeth=Zero
  S-R Flip-Flop1 : simulink_extras/Flip Flops/S-R Flip-Flop  initial_condition=0
  Subsystem1 : Subsystem
  Subsystem3 : Subsystem
  S_Limited : Outport  VectorParamsAs1DForOutWhenUnconnected=off
  !S_Limited : Outport  Port=2  VectorParamsAs1DForOutWhenUnconnected=off
  wires:
  S-R Flip-Flop1/1 -> S_Limited/1, Subsystem3/1(Sig)
  Product2/1 -> Data Type Conversion2/1
  Subsystem3/1(Trig) -> Product2/1
  Data Type Conversion2/1 -> S-R Flip-Flop1/1
  Data Type Conversion8/1 -> S-R Flip-Flop1/2
  Product3/1 -> Data Type Conversion8/1
  S-R Flip-Flop1/2 -> !S_Limited/1, Subsystem1/1(Sig)
  Subsystem1/1(Trig) -> Product3/2
  S/1 -> Product2/2
  !S/1 -> Product3/1

== system ac3_example_MMCT/Field-Oriented Control Induction Motor Drive/F.O.C./Detailed/Switching control/Control 3-4 ==
  S : Inport
  !S : Inport  Port=2
  Data Type Conversion2 : DataTypeConversion  OutDataTypeStr=boolean  SaturateOnIntegerOverflow=off  RndMeth=Floor
  Data Type Conversion8 : DataTypeConversion  OutDataTypeStr=boolean  SaturateOnIntegerOverflow=off  RndMeth=Floor
  Product2 : Product  RndMeth=Zero
  Product3 : Product  RndMeth=Zero
  S-R Flip-Flop1 : simulink_extras/Flip Flops/S-R Flip-Flop  initial_condition=0
  Subsystem1 : Subsystem
  Subsystem3 : Subsystem
  S_Limited : Outport  VectorParamsAs1DForOutWhenUnconnected=off
  !S_Limited : Outport  Port=2  VectorParamsAs1DForOutWhenUnconnected=off
  wires:
  !S/1 -> Product3/1
  S/1 -> Product2/2
  Subsystem1/1(Trig) -> Product3/2
  S-R Flip-Flop1/2 -> Subsystem1/1(Sig), !S_Limited/1
  Product3/1 -> Data Type Conversion8/1
  Data Type Conversion8/1 -> S-R Flip-Flop1/2
  Data Type Conversion2/1 -> S-R Flip-Flop1/1
  Subsystem3/1(Trig) -> Product2/1
  Product2/1 -> Data Type Conversion2/1
  S-R Flip-Flop1/1 -> Subsystem3/1(Sig), S_Limited/1

== system ac3_example_MMCT/Field-Oriented Control Induction Motor Drive/F.O.C./Detailed/Switching control/Control 5-6 ==
  S : Inport
  !S : Inport  Port=2
  Data Type Conversion2 : DataTypeConversion  OutDataTypeStr=boolean  SaturateOnIntegerOverflow=off  RndMeth=Floor
  Data Type Conversion8 : DataTypeConversion  OutDataTypeStr=boolean  SaturateOnIntegerOverflow=off  RndMeth=Floor
  Product2 : Product  RndMeth=Zero
  Product3 : Product  RndMeth=Zero
  S-R Flip-Flop1 : simulink_extras/Flip Flops/S-R Flip-Flop  initial_condition=0
  Subsystem1 : Subsystem
  Subsystem3 : Subsystem
  S_Limited : Outport  VectorParamsAs1DForOutWhenUnconnected=off
  !S_Limited : Outport  Port=2  VectorParamsAs1DForOutWhenUnconnected=off
  wires:
  S-R Flip-Flop1/1 -> S_Limited/1, Subsystem3/1(Sig)
  Product2/1 -> Data Type Conversion2/1
  Subsystem3/1(Trig) -> Product2/1
  Data Type Conversion2/1 -> S-R Flip-Flop1/1
  Data Type Conversion8/1 -> S-R Flip-Flop1/2
  Product3/1 -> Data Type Conversion8/1
  S-R Flip-Flop1/2 -> !S_Limited/1, Subsystem1/1(Sig)
  Subsystem1/1(Trig) -> Product3/2
  S/1 -> Product2/2
  !S/1 -> Product3/1

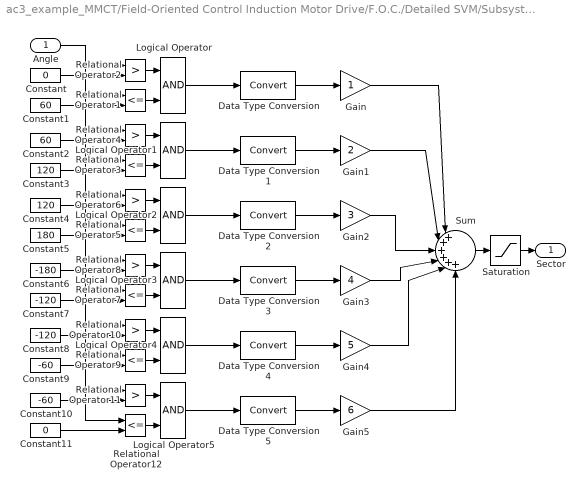
== system ac3_example_MMCT/Field-Oriented Control Induction Motor Drive/F.O.C./Detailed SVM/Subsystem1/ab vector sector ==
  Angle : Inport
  Constant : Constant  Value=0
  Constant1 : Constant  Value=60
  Constant10 : Constant  Value=-60
  Constant11 : Constant  Value=0
  Constant2 : Constant  Value=60
  Constant3 : Constant  Value=120
  Constant4 : Constant  Value=120
  Constant5 : Constant  Value=180
  Constant6 : Constant  Value=-180
  Constant7 : Constant  Value=-120
  Constant8 : Constant  Value=-120
  Constant9 : Constant  Value=-60
  Data Type Conversion{,1..5} (6 alike) : DataTypeConversion
  Gain : Gain  SaturateOnIntegerOverflow=on  OutDataTypeStr=Inherit: Same as input  ParamDataTypeStr=Inherit: Same as input
  Gain1 : Gain  Gain=2  SaturateOnIntegerOverflow=on  OutDataTypeStr=Inherit: Same as input  ParamDataTypeStr=Inherit: Same as input
  Gain2 : Gain  Gain=3  SaturateOnIntegerOverflow=on  OutDataTypeStr=Inherit: Same as input  ParamDataTypeStr=Inherit: Same as input
  Gain3 : Gain  Gain=4  SaturateOnIntegerOverflow=on  OutDataTypeStr=Inherit: Same as input  ParamDataTypeStr=Inherit: Same as input
  Gain4 : Gain  Gain=5  SaturateOnIntegerOverflow=on  OutDataTypeStr=Inherit: Same as input  ParamDataTypeStr=Inherit: Same as input
  Gain5 : Gain  Gain=6  SaturateOnIntegerOverflow=on  OutDataTypeStr=Inherit: Same as input  ParamDataTypeStr=Inherit: Same as input
  Logical Operator{,1..5} (6 alike) : Logic
  Relational Operator{1,3,5,7,9,12} (6 alike) : RelationalOperator  Operator=<=
  Relational Operator{2,4,6,8,10..11} (6 alike) : RelationalOperator  Operator=>
  Saturation : Saturate  UpperLimit=6  LowerLimit=1
  Sum : Sum  Inputs=|++++++  InputSameDT=on  SaturateOnIntegerOverflow=on  OutDataTypeStr=Inherit: Same as first input
  Sector : Outport  VectorParamsAs1DForOutWhenUnconnected=off
  wires:
  Saturation/1 -> Sector/1
  Sum/1 -> Saturation/1
  Gain5/1 -> Sum/6
  Gain4/1 -> Sum/5
  Gain3/1 -> Sum/4
  Gain2/1 -> Sum/3
  Gain1/1 -> Sum/2
  Gain/1 -> Sum/1
  Constant11/1 -> Relational Operator12/2
  Constant10/1 -> Relational Operator11/2
  Logical Operator5/1 -> Data Type Conversion5/1
  Relational Operator12/1 -> Logical Operator5/2
  Relational Operator11/1 -> Logical Operator5/1
  Constant9/1 -> Relational Operator9/2
  Constant8/1 -> Relational Operator10/2
  Logical Operator4/1 -> Data Type Conversion4/1
  Relational Operator9/1 -> Logical Operator4/2
  Relational Operator10/1 -> Logical Operator4/1
  Constant7/1 -> Relational Operator7/2
  Constant6/1 -> Relational Operator8/2
  Logical Operator3/1 -> Data Type Conversion3/1
  Relational Operator7/1 -> Logical Operator3/2
  Relational Operator8/1 -> Logical Operator3/1
  Constant5/1 -> Relational Operator5/2
  Constant4/1 -> Relational Operator6/2
  Logical Operator2/1 -> Data Type Conversion2/1
  Relational Operator5/1 -> Logical Operator2/2
  Relational Operator6/1 -> Logical Operator2/1
  Constant3/1 -> Relational Operator3/2
  Constant2/1 -> Relational Operator4/2
  Logical Operator1/1 -> Data Type Conversion1/1
  Relational Operator3/1 -> Logical Operator1/2
  Relational Operator4/1 -> Logical Operator1/1
  Constant1/1 -> Relational Operator1/2
  Constant/1 -> Relational Operator2/2
  Angle/1 -> Relational Operator12/1, Relational Operator11/1, Relational Operator9/1, Relational Operator10/1, Relational Operator7/1, Relational Operator8/1, Relational Operator5/1, Relational Operator6/1, Relational Operator3/1, Relational Operator4/1, Relational Operator1/1, Relational Operator2/1
  Logical Operator/1 -> Data Type Conversion/1
  Relational Operator1/1 -> Logical Operator/2
  Relational Operator2/1 -> Logical Operator/1
  Data Type Conversion/1 -> Gain/1
  Data Type Conversion1/1 -> Gain1/1
  Data Type Conversion2/1 -> Gain2/1
  Data Type Conversion3/1 -> Gain3/1
  Data Type Conversion4/1 -> Gain4/1
  Data Type Conversion5/1 -> Gain5/1

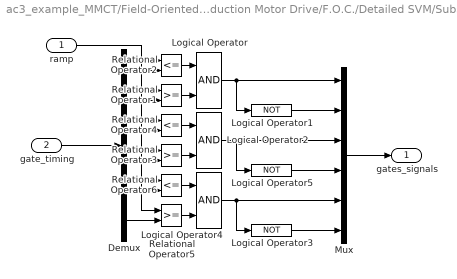
== system ac3_example_MMCT/Field-Oriented Control Induction Motor Drive/F.O.C./Detailed SVM/Subsystem1/gates logic1 ==
  ramp : Inport
  gate_timing : Inport  Port=2
  Demux : Demux  Outputs=6
      settings: DisplayOption=none
  Logical Operator : Logic
  Logical Operator1 : Logic  Operator=NOT
  Logical Operator2 : Logic
  Logical Operator3 : Logic  Operator=NOT
  Logical Operator4 : Logic
  Logical Operator5 : Logic  Operator=NOT
  Mux : Mux  Inputs=6
  Relational Operator1 : RelationalOperator
  Relational Operator2 : RelationalOperator  Operator=<=
  Relational Operator3 : RelationalOperator
  Relational Operator4 : RelationalOperator  Operator=<=
  Relational Operator5 : RelationalOperator
  Relational Operator6 : RelationalOperator  Operator=<=
  gates_signals : Outport  VectorParamsAs1DForOutWhenUnconnected=off
  wires:
  ramp/1 -> Relational Operator2/1, Relational Operator1/1, Relational Operator4/1, Relational Operator3/1, Relational Operator6/1, Relational Operator5/1
  Relational Operator2/1 -> Logical Operator/1
  Relational Operator1/1 -> Logical Operator/2
  Mux/1 -> gates_signals/1
  Relational Operator4/1 -> Logical Operator2/1
  Relational Operator3/1 -> Logical Operator2/2
  Relational Operator6/1 -> Logical Operator4/1
  Relational Operator5/1 -> Logical Operator4/2
  Logical Operator/1 -> Logical Operator1/1, Mux/1
  Logical Operator1/1 -> Mux/2
  Logical Operator2/1 -> Logical Operator5/1, Mux/3
  Logical Operator5/1 -> Mux/4
  Logical Operator4/1 -> Logical Operator3/1, Mux/5
  Logical Operator3/1 -> Mux/6
  Demux/1 -> Relational Operator2/2
  Demux/6 -> Relational Operator5/2
  Demux/5 -> Relational Operator6/2
  Demux/4 -> Relational Operator3/2
  Demux/3 -> Relational Operator4/2
  Demux/2 -> Relational Operator1/2
  gate_timing/1 -> Demux/1

== system ac3_example_MMCT/Field-Oriented Control Induction Motor Drive/F.O.C./Detailed SVM/Subsystem1/switching time calculator ==
  Trig : Inport
  Sector : Inport  Port=2
  a_b_vbus : Inport  Port=3
  Mux : Mux  Inputs=6
  switching_timing BrA : Subsystem  TreatAsAtomicUnit=on
  switching_timing BrB : Subsystem  TreatAsAtomicUnit=on
  switching_timing BrC : Subsystem  TreatAsAtomicUnit=on
  Gate timing : Outport  VectorParamsAs1DForOutWhenUnconnected=off
  wires:
  switching_timing BrA/1(L_off) -> Mux/1
  switching_timing BrA/2(L_on) -> Mux/2
  switching_timing BrB/1(L_off) -> Mux/3
  switching_timing BrB/2(L_on) -> Mux/4
  switching_timing BrC/1(L_off) -> Mux/5
  switching_timing BrC/2(L_on) -> Mux/6
  Sector/1 -> switching_timing BrB/1(sector), switching_timing BrC/1(sector), switching_timing BrA/1(sector)
  a_b_vbus/1 -> switching_timing BrB/2(Vab_inp), switching_timing BrA/2(vab_in), switching_timing BrC/2(Vab_inp)
  Trig/1 -> switching_timing BrA/Trigger, switching_timing BrB/Trigger, switching_timing BrC/Trigger
  Mux/1 -> Gate timing/1

== system ac3_example_MMCT/Field-Oriented Control Induction Motor Drive/F.O.C./Detailed SVM/Subsystem2/Subsystem ==
  Q : Inport
  Q1 : Inport  Port=2
  Math Function : Math  Operator=reciprocal
  PID Controller : slpidlib/PID Controller  Controller=PID  Form=Parallel  TimeDomain=Continuous-time  UseExternalTs=off  SampleTime=-1  IntegratorMethod=Forward Euler  FilterMethod=Forward Euler  ControllerParametersSource=internal  P=1  I=1  UseKiTs=off  D=0  N=100  UseFilter=on  TunerSelectOption=Transfer Function Based (PID Tuner App)  InitialConditionSource=internal  InitialConditionForIntegrator=0  InitialConditionForFilter=0  DifferentiatorICPrevScaledInput=0  ExternalReset=none  TrackingMode=off  Kt=1  LimitOutput=off  SatLimitsSource=internal  UpperSaturationLimit=inf  LowerSaturationLimit=-inf  LinearizeAsGain=on  AntiWindupMode=none  Kb=1  LimitIntegrator=off  UpperIntegratorSaturationLimit=inf  LowerIntegratorSaturationLimit=-inf  POutMin=[]  POutMax=[]  IOutMin=[]  IOutMax=[]  DOutMin=[]  DOutMax=[]  NOutMin=[]  NOutMax=[]  SumOutMin=[]  SumOutMax=[]  SaturationOutMin=[]  SaturationOutMax=[]  PParamMin=[]  PParamMax=[]  IParamMin=[]  IParamMax=[]  DParamMin=[]  DParamMax=[]  NParamMin=[]  NParamMax=[]  KbParamMin=[]  KbParamMax=[]  KtParamMin=[]  KtParamMax=[]  KbOutMin=[]  KbOutMax=[]  KtOutMin=[]  KtOutMax=[]  IntegratorOutMin=[]  IntegratorOutMax=[]  FilterOutMin=[]  FilterOutMax=[]  SumI1OutMin=[]  SumI1OutMax=[]  SumI2OutMin=[]  SumI2OutMax=[]  SumI3OutMin=[]  SumI3OutMax=[]  SumI4OutMin=[]  SumI4OutMax=[]  SumDOutMin=[]  SumDOutMax=[]  DifferentiatorOutMin=[]  DifferentiatorOutMax=[]  FilterDiffOutCoefMin=[]  FilterDiffOutCoefMax=[]  ReciprocalOutMin=[]  ReciprocalOutMax=[]  SumDenOutMin=[]  SumDenOutMax=[]  SumNumOutMin=[]  SumNumOutMax=[]  DivideOutMin=[]  DivideOutMax=[]  UdiffTsProdOutMin=[]  UdiffTsProdOutMax=[]  NTsProdOutMin=[]  NTsProdOutMax=[]  UintegralTsProdOutMin=[]  UintegralTsProdOutMax=[]  UngainTsProdOutMin=[]  UngainTsProdOutMax=[]  ClampingZeroOutDataTypeStr=Inherit: Inherit via back propagation  ClampingZeroOutMin=[]  ClampingZeroOutMax=[]  FilterDenConstantOutDataTypeStr=Inherit: Inherit via back propagation  FilterDenConstantOutMin=[]  FilterDenConstantOutMax=[]  PCopyOutDataTypeStr=Inherit: Inherit via back propagation  PCopyOutMin=[]  PCopyOutMax=[]  NCopyOutDataTypeStr=Inherit: Inherit via back propagation  NCopyOutMin=[]  NCopyOutMax=[]  IntegratorContinuousStateAttributes=''  IntegratorStateMustResolveToSignalObject=off  IntegratorRTWStateStorageClass=Auto  FilterContinuousStateAttributes=''  FilterStateMustResolveToSignalObject=off  FilterRTWStateStorageClass=Auto  ParallelPVariant=InternalParameters  IdealPVariant=Disabled  IVariant=InternalParameters  DVariant=InternalParameters  IntegratorVariant=Continuous  SatVariant=Disabled  AWVariant=Passthrough  PCopyVariant=Disabled  TRVariant=Disabled  FdbkBlocksVariant=Forward  IdealPFdbkVariant=Disabled  SatFdbkVariant=Disabled  DerivativeFilterVariant=ContFilter  NVariant=InternalParameters  NCopyVariant=Disabled  FilterICVariant=InternalICsFilter  IntegratorICVariant=InternalICs  ExternalResetVariant=Disabled  TRSumVariant=Passthrough  SumFdbkVariant=Disabled  SumVariant=Sum_PID  TsampFilterVariant=InternalTs  TsampNgainVariant=Passthrough  TsampIntegralVariant=Disabled_SignalSpec  ExternalSaturationOutDataTypeStr=Inherit: Same as second input
  Sum : Sum  Inputs=|++
  Tr : Outport
  wires:
  PID Controller/1 -> Math Function/1
  Sum/1 -> PID Controller/1
  Q1/1 -> Sum/2
  Math Function/1 -> Tr/1  "Tr"
  Q/1 -> Sum/1

== system ac3_example_MMCT/Field-Oriented Control Induction Motor Drive/F.O.C./Detailed SVM/dq//ab1/DQ-ABC ==
  Vq* : Inport
  Vd* : Inport  Port=2
  Teta : Inport  Port=3
  Fcn : Fcn  Expr=sin(u)
  Fcn1 : Fcn  Expr=cos(u)
  Gain2 : Gain  SaturateOnIntegerOverflow=on  OutDataTypeStr=Inherit: Same as input  ParamDataTypeStr=Inherit: Same as input
  Gain3 : Gain  SaturateOnIntegerOverflow=on  OutDataTypeStr=Inherit: Same as input  ParamDataTypeStr=Inherit: Same as input
  Gain4 : Gain  SaturateOnIntegerOverflow=on  OutDataTypeStr=Inherit: Same as input  ParamDataTypeStr=Inherit: Same as input
  Mux : Mux
  Mux2 : Mux  Inputs=3
  ia : Fcn  Expr=u[3]*u[1] + u[4]*u[2]
  ib : Fcn  Expr=(-u[2]-1.7320508*u[1])*u[4]*0.5+(-u[1]+1.7320508*u[2])*u[3]*0.5
  ic : Sum  Inputs=--  InputSameDT=on  SaturateOnIntegerOverflow=on  OutDataTypeStr=Inherit: Same as first input
  Vabc* : Outport  InitialOutput=0  VectorParamsAs1DForOutWhenUnconnected=off
  wires:
  Fcn/1 -> Mux/2
  Fcn1/1 -> Mux/1
  Mux2/1 -> Vabc*/1
  Mux/1 -> ib/1, ia/1
  Teta/1 -> Fcn1/1, Fcn/1
  Vq*/1 -> Mux/3
  Vd*/1 -> Mux/4
  Gain3/1 -> Mux2/2
  ic/1 -> Gain4/1
  Gain4/1 -> Mux2/3
  Gain2/1 -> Mux2/1
  ia/1 -> Gain2/1, ic/2
  ib/1 -> Gain3/1, ic/1

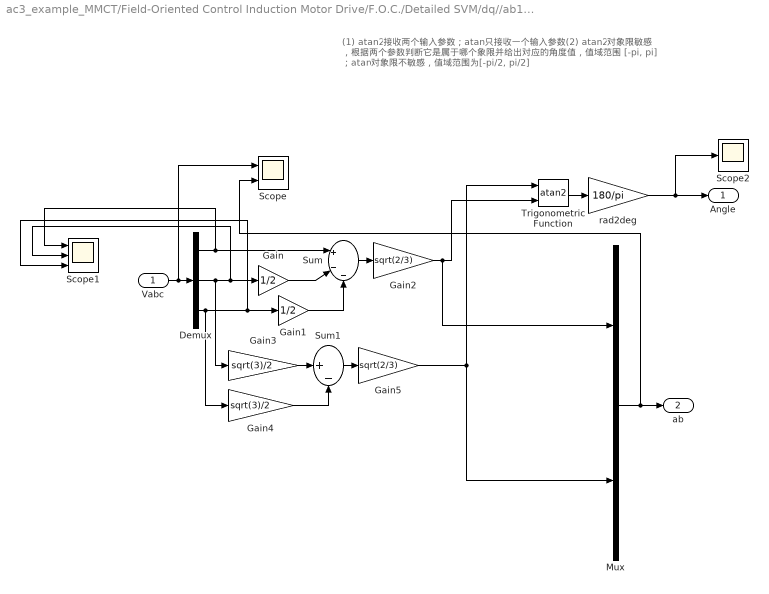
== system ac3_example_MMCT/Field-Oriented Control Induction Motor Drive/F.O.C./Detailed SVM/dq//ab1/ab transform ==
  note: (1) atan2接收两个输入参数；atan只接收一个输入参数(2) atan2对象限敏感 ，根据两个参数判断它是属于哪个象限并给出对应的角度值，值域范围 [-pi, pi] ；atan对象限不敏感，值域范围为[-pi/2, pi/2]
  Vabc : Inport
  Demux : Demux  Outputs=3
      settings: DisplayOption=none
  Gain : Gain  Gain=1/2  SaturateOnIntegerOverflow=on  OutDataTypeStr=Inherit: Same as input  ParamDataTypeStr=Inherit: Same as input
  Gain1 : Gain  Gain=1/2  SaturateOnIntegerOverflow=on  OutDataTypeStr=Inherit: Same as input  ParamDataTypeStr=Inherit: Same as input
  Gain2 : Gain  Gain=sqrt(2/3)  SaturateOnIntegerOverflow=on  OutDataTypeStr=Inherit: Same as input  ParamDataTypeStr=Inherit: Same as input
  Gain3 : Gain  Gain=sqrt(3)/2  SaturateOnIntegerOverflow=on  OutDataTypeStr=Inherit: Same as input  ParamDataTypeStr=Inherit: Same as input
  Gain4 : Gain  Gain=sqrt(3)/2  SaturateOnIntegerOverflow=on  OutDataTypeStr=Inherit: Same as input  ParamDataTypeStr=Inherit: Same as input
  Gain5 : Gain  Gain=sqrt(2/3)  SaturateOnIntegerOverflow=on  OutDataTypeStr=Inherit: Same as input  ParamDataTypeStr=Inherit: Same as input
  Mux : Mux  Inputs=2
  Scope : Scope  NumInputPorts=2
  Scope1 : Scope  NumInputPorts=3
  Scope2 : Scope
  Sum : Sum  Inputs=|+--  InputSameDT=on  SaturateOnIntegerOverflow=on  OutDataTypeStr=Inherit: Same as first input
  Sum1 : Sum  Inputs=|+-  InputSameDT=on  SaturateOnIntegerOverflow=on  OutDataTypeStr=Inherit: Same as first input
  Trigonometric Function : Trigonometry  Operator=atan2
  rad2deg : Gain  Gain=180/pi  SaturateOnIntegerOverflow=on  OutDataTypeStr=Inherit: Same as input  ParamDataTypeStr=Inherit: Same as input
  Angle : Outport  VectorParamsAs1DForOutWhenUnconnected=off
  ab : Outport  Port=2  VectorParamsAs1DForOutWhenUnconnected=off
  wires:
  Demux/3 -> Scope1/3, Gain1/1, Gain4/1
  Demux/2 -> Scope1/2, Gain/1, Gain3/1
  Demux/1 -> Scope1/1, Sum/1
  Vabc/1 -> Scope/1, Demux/1
  rad2deg/1 -> Scope2/1, Angle/1
  Gain/1 -> Sum/2
  Gain5/1 -> Mux/2, Trigonometric Function/1
  Mux/1 -> Scope/2, ab/1
  Trigonometric Function/1 -> rad2deg/1
  Gain1/1 -> Sum/3
  Sum/1 -> Gain2/1
  Sum1/1 -> Gain5/1
  Gain4/1 -> Sum1/2
  Gain3/1 -> Sum1/1
  Gain2/1 -> Mux/1, Trigonometric Function/2

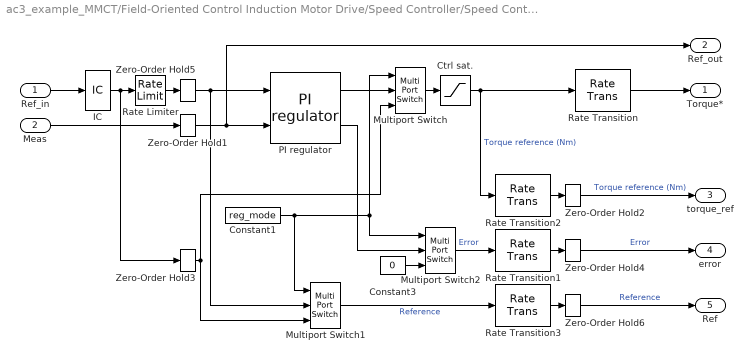
== system ac3_example_MMCT/Field-Oriented Control Induction Motor Drive/Speed Controller/Speed Controller (AC)/AC345/Speed controller (generic AC) ==
  Ref_in : Inport
  Meas : Inport  Port=2
  Constant1 : Constant  Value=reg_mode
  Constant3 : Constant  Value=0
  Ctrl sat. : Saturate  UpperLimit=ctrl_sat(2)  LowerLimit=ctrl_sat(1)
  IC : InitialCondition  Value=0
  Multiport Switch : MultiPortSwitch  Inputs=2  InputSameDT=off
  Multiport Switch1 : MultiPortSwitch  Inputs=2  InputSameDT=off
  Multiport Switch2 : MultiPortSwitch  Inputs=2  InputSameDT=off
  PI regulator : spsDrivesPrivateModels/PI regulator  kp=kp  ki=ki  fc=fc  out_sat=ctrl_sat  Tsc=Tsc
  Rate Limiter : RateLimiter  RisingSlewLimit=ramp(2)  FallingSlewLimit=ramp(1)  LinearizeAsGain=off
  Rate Transition{,1..3} (4 alike) : RateTransition
  Zero-Order Hold1 : ZeroOrderHold  SampleTime=Tsc
  Zero-Order Hold2 : ZeroOrderHold  SampleTime=Ts
  Zero-Order Hold3 : ZeroOrderHold  SampleTime=Tsc
  Zero-Order Hold4 : ZeroOrderHold  SampleTime=Ts
  Zero-Order Hold5 : ZeroOrderHold  SampleTime=Tsc
  Zero-Order Hold6 : ZeroOrderHold  SampleTime=Ts
  Torque* : Outport  VectorParamsAs1DForOutWhenUnconnected=off
  Ref_out : Outport  Port=2  VectorParamsAs1DForOutWhenUnconnected=off
  torque_ref : Outport  Port=3  VectorParamsAs1DForOutWhenUnconnected=off
  error : Outport  Port=4  VectorParamsAs1DForOutWhenUnconnected=off
  Ref : Outport  Port=5  VectorParamsAs1DForOutWhenUnconnected=off
  wires:
  Zero-Order Hold6/1 -> Ref/1  "Reference"
  Zero-Order Hold4/1 -> error/1  "Error"
  Zero-Order Hold2/1 -> torque_ref/1  "Torque reference (Nm)"
  Rate Transition3/1 -> Zero-Order Hold6/1
  Rate Transition1/1 -> Zero-Order Hold4/1
  PI regulator/1 -> Multiport Switch/2
  PI regulator/2 -> Multiport Switch2/2
  Multiport Switch2/1 -> Rate Transition1/1  "Error"
  Multiport Switch1/1 -> Rate Transition3/1  "Reference"
  Zero-Order Hold5/1 -> Multiport Switch1/2, PI regulator/1
  Zero-Order Hold1/1 -> Ref_out/1, PI regulator/2
  Multiport Switch/1 -> Ctrl sat./1
  IC/1 -> Rate Limiter/1, Zero-Order Hold3/1
  Constant1/1 -> Multiport Switch2/1, Multiport Switch/1, Multiport Switch1/1
  Ctrl sat./1 -> Rate Transition/1, Rate Transition2/1  "Torque reference (Nm)"
  Rate Transition/1 -> Torque*/1
  Rate Limiter/1 -> Zero-Order Hold5/1
  Rate Transition2/1 -> Zero-Order Hold2/1
  Zero-Order Hold3/1 -> Multiport Switch/3, Multiport Switch1/3
  Constant3/1 -> Multiport Switch2/3
  Ref_in/1 -> IC/1
  Meas/1 -> Zero-Order Hold1/1
